simulink model "chap11_01_10_mdl"  (R2013b)
settings: Solver=ode45  StartTime=0.0  StopTime=10.0  RelTol=1e-3
InitFcn:
  | a = 1;
  | b = 0.3;
settings Model: Creator=Administrator  LastModifiedBy=sunzx.fnst

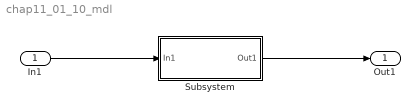
== system chap11_01_10_mdl ==
  In1 : Inport
  Subsystem : Subsystem
      mask Display:
      | color('red');
      | text(0, 0, 'y = a * x^2 + b', 'horizontalAlignment', 'left', 'verticalAlignment', 'bottom')
  Out1 : Outport
  wires:
  In1/1 -> Subsystem/1(In1)
  Subsystem/1(Out1) -> Out1/1

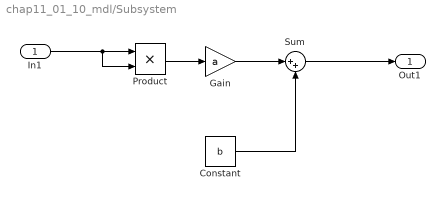
== system chap11_01_10_mdl/Subsystem ==
  In1 : Inport
  Constant : Constant  Value=b
  Gain : Gain  Gain=a
  Product : Product
  Sum : Sum  Inputs=|++
  Out1 : Outport
  wires:
  Gain/1 -> Sum/1
  Constant/1 -> Sum/2
  In1/1 -> Product/2, Product/1
  Sum/1 -> Out1/1
  Product/1 -> Gain/1
